simulink model "Mesh_Analysis"  (R2024b)
settings: Solver=VariableStepAuto  StartTime=0.0  StopTime=10.0  RelTol=1e-3
libraries: spsSeriesRLCBranchLib x14, spsCurrentMeasurementLib x10, spsControlledCurrentSourceLib x9, spsVoltageMeasurementLib x5, spsDCVoltageSourceLib x4, spsACVoltageSourceLib x1, sps_lib x1
settings Model: Creator=priya  LastModifiedBy=priya

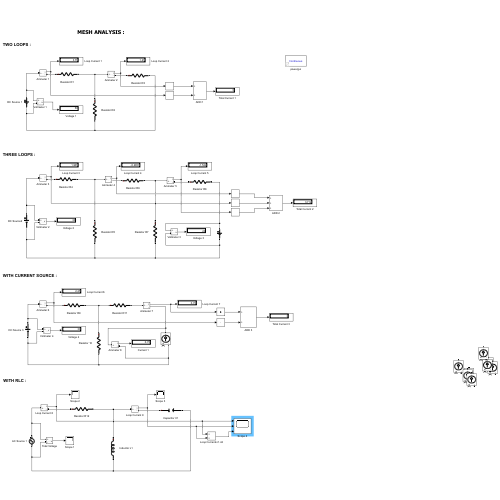
[thumbnail: Simulink's stored preview of the top-level diagram]
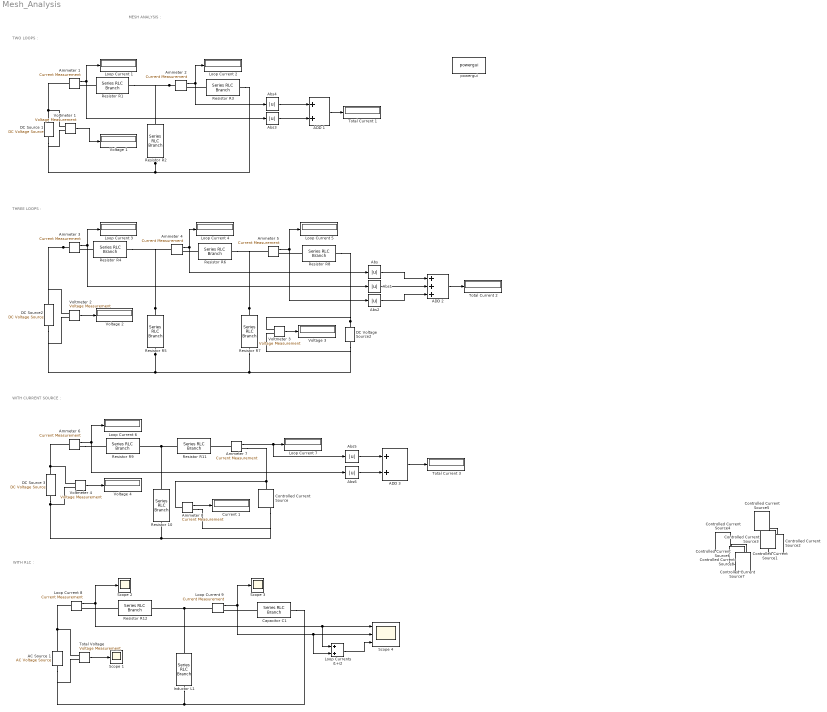
== system Mesh_Analysis ==
  note: WITH RLC :
  note: THREE LOOPS :
  note: MESH ANALYSIS :
  note: TWO LOOPS :
  note: WITH CURRENT SOURCE :
  AC Source 1 : spsACVoltageSourceLib/AC Voltage Source  Amplitude=50  Phase=0  Frequency=60  SampleTime=0  Measurements=None  BusType=swing  Pref=10e3  Qref=0  Qmin=-inf  Qmax=+inf
  ADD 1 : Sum
  ADD 2 : Sum  Inputs=+++
  ADD 3 : Sum
  Abs{,1..6} (7 alike) : Abs  SaturateOnIntegerOverflow=off
  Ammeter {1..8} (8 alike) : spsCurrentMeasurementLib/Current Measurement  PhasorSimulation=off  OutputType=Complex  PSBequivalent=0
  Capacitor C1 : spsSeriesRLCBranchLib/Series RLC Branch  LConnTagsString=__new0  RConnTagsString=__new0  BranchType=C  Resistance=10  Inductance=1e-3  SetiL0=off  InitialCurrent=0  Capacitance=10  Setx0=off  InitialVoltage=0  Measurements=None
  Controlled Current Source{,1..8} (9 alike) : spsControlledCurrentSourceLib/Controlled Current Source  Initialize=on  Source_Type=DC  Amplitude=10  Phase=0  Frequency=0  Measurements=Current
  Current 1 : Display
  DC Source 1 : spsDCVoltageSourceLib/DC Voltage Source  Amplitude=50  Measurements=None
  DC Source 3 : spsDCVoltageSourceLib/DC Voltage Source  Amplitude=30  Measurements=None
  DC Source2 : spsDCVoltageSourceLib/DC Voltage Source  Amplitude=30  Measurements=None
  DC Voltage Source2 : spsDCVoltageSourceLib/DC Voltage Source  Amplitude=20  Measurements=None
  Inductor L1 : spsSeriesRLCBranchLib/Series RLC Branch  LConnTagsString=__new0  RConnTagsString=__new0  BranchType=L  Resistance=10  Inductance=10  SetiL0=off  InitialCurrent=0  Capacitance=1e-6  Setx0=off  InitialVoltage=0  Measurements=None
  Loop Current {1..6} (6 alike) : Display
  "Loop Current 7 " : Display
  Loop Current 8 : spsCurrentMeasurementLib/Current Measurement  PhasorSimulation=off  OutputType=Complex  PSBequivalent=0
  Loop Current 9 : spsCurrentMeasurementLib/Current Measurement  PhasorSimulation=off  OutputType=Complex  PSBequivalent=0
  Loop Currents i1+i2 : Sum
  Resistor 10 : spsSeriesRLCBranchLib/Series RLC Branch  LConnTagsString=__new0  RConnTagsString=__new0  BranchType=R  Resistance=5  Inductance=1e-3  SetiL0=off  InitialCurrent=0  Capacitance=1e-6  Setx0=off  InitialVoltage=0  Measurements=None
  Resistor R{1,3..4,7,9,11..12} (7 alike) : spsSeriesRLCBranchLib/Series RLC Branch  LConnTagsString=__new0  RConnTagsString=__new0  BranchType=R  Resistance=10  Inductance=1e-3  SetiL0=off  InitialCurrent=0  Capacitance=1e-6  Setx0=off  InitialVoltage=0  Measurements=None
  Resistor R{2,5..6,8} (4 alike) : spsSeriesRLCBranchLib/Series RLC Branch  LConnTagsString=__new0  RConnTagsString=__new0  BranchType=R  Resistance=5  Inductance=1e-3  SetiL0=off  InitialCurrent=0  Capacitance=1e-6  Setx0=off  InitialVoltage=0  Measurements=None
  Scope 1 : Scope
  Scope 2 : Scope
  Scope 3 : Scope
  Scope 4 : Scope  NumInputPorts=3
  Total Current 1 : Display
  Total Current 2 : Display
  Total Current 3 : Display
  Total Voltage : spsVoltageMeasurementLib/Voltage Measurement  PhasorSimulation=off  OutputType=Complex  PSBequivalent=0
  Voltage {1..4} (4 alike) : Display
  Voltmeter {1..4} (4 alike) : spsVoltageMeasurementLib/Voltage Measurement  PhasorSimulation=off  OutputType=Complex  PSBequivalent=0
  powergui : sps_lib/powergui  Priority=1  SimulationMode=Continuous  SampleTime=50e-6  frequency=60  Iterations=50  frequencyindice=0  Pbase=100e6  ErrMax=1e-4  UnitsV=kV  UnitsW=MW  buscounter=0  FunctionMessages=off  echomessages=off  EnableUseOfTLC=off  CurrentSourceSwitches=off  DisableSnubberDevices=off  DisableRonSwitches=off  DisableVfSwitches=off  DisplayEquations=off  AutomaticDiscreteSolvers=off  SolverType=Tustin/Backward Euler (TBE)  Interpol=off  ExternalGateDelay=off  methode=off  Ts=100  x0status=blocks  SPID=on  SwTol=0  HookPort=off  NonlinearTolerance=1e-4  nMaxIteration=100  ContinueOnMaxIteration=off  RestoreLinks=warning  ResistiveCurrentMeasurement=off  Frange=[0:2:500]  Ylog=off  Xlog=on  ShowGrid=off  save=off  variable=ZData  structure=0  ZoomFFT=off  StartTime=0.0  cycles=1  DisplayStyle=1  fundamental=60  FreqAxis=off  MaxFrequency=1000  frequencyindicesteady=1  RmsSteady=1  display=off
  wires:
  ADD 2/1 -> Total Current 2/1
  Abs/1 -> ADD 2/1
  Abs1/1 -> ADD 2/2
  Ammeter 4/1 -> Abs/1, Loop Current 4/1
  Voltmeter 3/1 -> Voltage 3/1
  Abs2/1 -> ADD 2/3
  Voltmeter 2/1 -> Voltage 2/1
  Ammeter 3/1 -> Abs1/1, Loop Current 3/1
  Ammeter 5/1 -> Abs2/1, Loop Current 5/1
  Ammeter 1/1 -> Abs3/1, Loop Current 1/1
  Voltmeter 1/1 -> Voltage 1/1
  Ammeter 2/1 -> Abs4/1, Loop Current 2/1
  Abs4/1 -> ADD 1/1
  Abs3/1 -> ADD 1/2
  ADD 1/1 -> Total Current 1/1
  Ammeter 6/1 -> Abs6/1, Loop Current 6/1
  Voltmeter 4/1 -> Voltage 4/1
  Ammeter 8/1 -> Current 1/1
  Ammeter 7/1 -> Abs5/1, "Loop Current 7 "/1
  Abs5/1 -> ADD 3/1
  Abs6/1 -> ADD 3/2
  ADD 3/1 -> Total Current 3/1
  Loop Current 8/1 -> Loop Currents i1+i2/1, Scope 4/1, Scope 2/1
  Total Voltage/1 -> Scope 1/1
  Loop Current 9/1 -> Loop Currents i1+i2/2, Scope 4/2, Scope 3/1
  Loop Currents i1+i2/1 -> Scope 4/3
  connections:
  Resistor R5/LConn1 -- Resistor R4/RConn1 -- Ammeter 4/LConn1
  Ammeter 3/LConn1 -- DC Source2/RConn1 -- Voltmeter 2/LConn1
  Resistor R5/RConn1 -- DC Source2/LConn1 -- Voltmeter 2/LConn2 -- Resistor R7/RConn1 -- DC Voltage Source2/LConn1 -- Voltmeter 3/LConn2
  Resistor R7/LConn1 -- Resistor R6/RConn1 -- Ammeter 5/LConn1
  DC Voltage Source2/RConn1 -- Resistor R8/RConn1 -- Voltmeter 3/LConn1
  Resistor R6/LConn1 -- Ammeter 4/RConn1
  Resistor R8/LConn1 -- Ammeter 5/RConn1
  Resistor R4/LConn1 -- Ammeter 3/RConn1
  Ammeter 2/LConn1 -- Resistor R1/RConn1 -- Resistor R2/LConn1
  Ammeter 1/LConn1 -- DC Source 1/RConn1 -- Voltmeter 1/LConn1
  Resistor R2/RConn1 -- Voltmeter 1/LConn2 -- DC Source 1/LConn1 -- Resistor R3/RConn1
  Resistor R3/LConn1 -- Ammeter 2/RConn1
  Resistor R1/LConn1 -- Ammeter 1/RConn1
  Ammeter 6/RConn1 -- Resistor R9/LConn1
  Ammeter 6/LConn1 -- DC Source 3/RConn1 -- Voltmeter 4/LConn1
  Resistor 10/LConn1 -- Resistor R11/LConn1 -- Resistor R9/RConn1
  DC Source 3/LConn1 -- Voltmeter 4/LConn2 -- Ammeter 8/RConn1 -- Controlled Current Source/LConn1 -- Resistor 10/RConn1
  Ammeter 8/LConn1 -- Ammeter 7/RConn1 -- Controlled Current Source/RConn1
  Ammeter 7/LConn1 -- Resistor R11/RConn1
  Total Voltage/LConn1 -- AC Source 1/RConn1 -- Loop Current 8/LConn1
  Resistor R12/LConn1 -- Loop Current 8/RConn1
  Loop Current 9/LConn1 -- Inductor L1/LConn1 -- Resistor R12/RConn1
  Capacitor C1/RConn1 -- AC Source 1/LConn1 -- Total Voltage/LConn2 -- Inductor L1/RConn1
  Capacitor C1/LConn1 -- Loop Current 9/RConn1
